simulink model "Simulink"  (R2014a)
settings: Solver=ode45  StartTime=0.0  StopTime=70  RelTol=1e-3
values from neighbouring files (symbols this model uses):
  K = [-4.2029e-03 -3.4474e-01 -1.5683e-01 0.0000 -1.0000e-02]    [Initiallize.m]
  quat0 = attitude(ROCKET.azimth, ROCKET.elevation)'    [Initiallize.m]    (also in RocketSim.m = attitude(azimth, elevation); params.m = attitude(azimth, elevation); params_M3S.m = attitude(ROCKET.azimth, ROCKET.elevation))
  ROCKET = params_rocket()    [Initiallize.m]    (also in params_M3S.m = struct(  'm0', 45247.4,  'Isp', 266,  'g0', 9.80665,  'FT', )
  tau_delta = 0.5    [Initiallize.m]
  Tr = 0.0    (= 0)    [Initiallize.m]
  VWH = [0.0; 0.0; 0.0]    [Initiallize.m]    (also in params.m = [0; 0; 0]; params_M3S.m = [0; 0; 0]; rocket_dynamics.m = [0; 0; 0])
  x0 = [ROCKET.m0; ROCKET.pos0; ROCKET.vel0; quat0; ROCKET.omega0]    [Initiallize.m]    (also in RocketSim.m = [m0; pos0; vel0; quat0; omega0]; params.m = [m0; pos0; vel0; quat0; omega0]; params_M3S.m = [ROCKET.m0; pos0; vel0; quat0; omega0])
undefined symbols (not defined in the file or in its folder): angle0
settings Model: Creator=ikemoto  LastModifiedBy=ikemoto

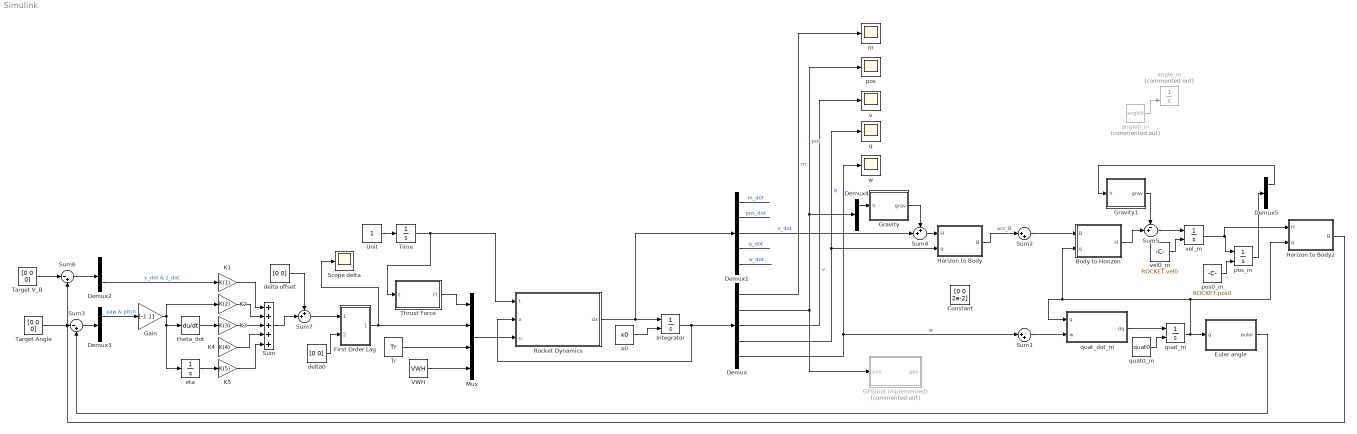
== system Simulink ==
  Body to Horizon : MATLAB Function  TreatAsAtomicUnit=on
  Constant : Constant  Value=[0 0 2e-2]
  Demux : Demux  Outputs=[1 3 3 4 3]
  Demux1 : Demux  Outputs=[1 3 3 4 3]
  Demux2 : Demux  Outputs=[1 2]
  Demux3 : Demux  Outputs=[2 1]
  Demux4 : Demux  Outputs=3
  Demux5 : Demux  Outputs=3
  Euler angle : MATLAB Function  TreatAsAtomicUnit=on
  First Order Lag : Subsystem
  GPS(not implemented) : MATLAB Function  Commented=on  TreatAsAtomicUnit=on
  Gain : Gain  Gain=[-1 1]
  Gravity : MATLAB Function  TreatAsAtomicUnit=on
  Gravity1 : MATLAB Function  TreatAsAtomicUnit=on
  Horizon to Body : MATLAB Function  TreatAsAtomicUnit=on
  Horizon to Body2 : MATLAB Function  TreatAsAtomicUnit=on
  Integrator : Integrator  InitialConditionSource=external  InitialCondition=[4.0 0.0 0.0 0.0 0.0 0.0 0.0 1.0 0.0 0.0 0.0 0.0 0.0 0.0]
  K1 : Gain  Gain=K(1)
  K2 : Gain  Gain=K(2)
  K3 : Gain  Gain=K(3)
  K4 : Gain  Gain=K(4)
  K5 : Gain  Gain=K(5)
  Mux : Mux  Inputs=[1 2 1 3]
  Rocket Dynamics : MATLAB Function  TreatAsAtomicUnit=on
  Scope delta : Scope
      settings: SaveName=ScopeData7
  Sum : Sum  Inputs=+++++
  Sum1 : Sum  Inputs=|++
  Sum2 : Sum  Inputs=|++
  Sum3 : Sum  Inputs=|-+
  Sum4 : Sum  Inputs=++|
  Sum5 : Sum  Inputs=-+|
  Sum6 : Sum  Inputs=|-+
  Sum7 : Sum  Inputs=++|
  Target Angle : Constant  Value=[0 0 0]
  Target V_B : Constant  Value=[0 0 0]
  Thrust Force : MATLAB Function  TreatAsAtomicUnit=on
  Time : Integrator
  Tr : Constant  Value=Tr
  Unit : Constant
  VWH : Constant  Value=VWH
  angle0_m : Constant  Commented=on  Value=angle0
  angle_m : Integrator  Commented=on  InitialConditionSource=external
  delta offset : Constant  Value=[0 0]
  delta0 : Constant  Value=[0 0]
  eta : Integrator
  m : Scope
  pos : Scope
  pos0_m : Constant  Value=ROCKET.pos0
  pos_m : Integrator  InitialConditionSource=external
  q : Scope
      settings: SaveName=ScopeData3
  quat0_m : Constant  Value=quat0
  quat_dot_m : MATLAB Function  TreatAsAtomicUnit=on
  quat_m : Integrator  InitialConditionSource=external
  theta_dot : Derivative
  v : Scope
      settings: SaveName=ScopeData2
  vel0_m : Constant  Value=ROCKET.vel0
  vel_m : Integrator  InitialConditionSource=external
  w : Scope
      settings: SaveName=ScopeData4
  x0 : Constant  Value=x0
  wires:
  Rocket Dynamics/1(dx) -> Demux1/1, Integrator/1
  Integrator/1 -> Rocket Dynamics/2(x), Demux/1
  x0/1 -> Integrator/2
  Demux/1 -> m/1  "m"
  Demux/2 -> pos/1, Demux4/1, GPS(not implemented)/1(pos)  "pos"
  Demux/3 -> v/1  "v"
  Time/1 -> Thrust Force/1(t), Rocket Dynamics/1(t)
  Unit/1 -> Time/1
  Demux1/1 -> ?  "m_dot"
  Demux1/2 -> ?  "pos_dot"
  Demux1/4 -> ?  "q_dot"
  Demux1/5 -> ?  "w_dot"
  Demux/5 -> w/1, Sum1/1  "w"
  Mux/1 -> Rocket Dynamics/3(u)
  VWH/1 -> Mux/4
  Tr/1 -> Mux/3
  vel_m/1 -> Horizon to Body2/1(H), pos_m/1
  eta/1 -> K5/1
  theta_dot/1 -> K3/1
  Gain/1 -> K2/1, eta/1, theta_dot/1
  quat_dot_m/1(dq) -> quat_m/1
  quat0_m/1 -> quat_m/2
  quat_m/1 -> Euler angle/1(q), quat_dot_m/1(q), Body to Horizon/2(q), Horizon to Body2/2(q)
  Thrust Force/1(Ft) -> Mux/1
  Sum1/1 -> quat_dot_m/2(w)
  ? -> Sum1/2  "error"
  ? -> Sum2/2  "error"
  angle0_m/1 -> angle_m/2
  Sum2/1 -> Body to Horizon/1(B)
  vel0_m/1 -> vel_m/2
  pos0_m/1 -> pos_m/2
  Euler angle/1(euler) -> Sum3/2
  Demux2/2 -> K1/1  "y_dot & z_dot"
  K2/1 -> Sum/2
  K1/1 -> Sum/1
  K3/1 -> Sum/3
  K4/1 -> Sum/4
  K5/1 -> Sum/5
  Demux/4 -> q/1, Horizon to Body/2(q)  "q"
  Horizon to Body2/1(B) -> Sum6/2
  Sum3/1 -> Demux3/1
  Target Angle/1 -> Sum3/1
  Demux3/1 -> Gain/1  "yaw & pitch"
  delta0/1 -> First Order Lag/2(delta0)
  First Order Lag/1(delta) -> Scope delta/1, Mux/2
  Horizon to Body/1(B) -> Sum2/1  "acc_B"
  Demux4/1 -> Gravity/1(h)
  Sum5/1 -> vel_m/1
  Body to Horizon/1(H) -> Sum5/2
  Gravity1/1(grav) -> Sum5/1
  pos_m/1 -> Demux5/1
  Demux5/1 -> Gravity1/1(h)
  Sum4/1 -> Horizon to Body/1(H)
  Gravity/1(grav) -> Sum4/1
  Demux1/3 -> Sum4/2  "v_dot"
  Sum6/1 -> Demux2/1
  Target V_B/1 -> Sum6/1
  Sum7/1 -> First Order Lag/1(delta_i)
  Sum/1 -> Sum7/2
  delta offset/1 -> Sum7/1

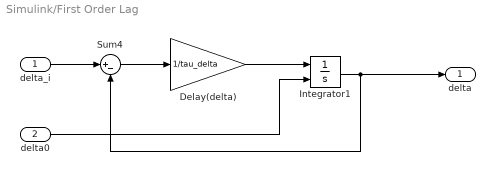
== system Simulink/First Order Lag ==
  delta_i : Inport
  delta0 : Inport  Port=2
  Delay(delta) : Gain  Gain=1/tau_delta
  Integrator1 : Integrator  InitialConditionSource=external  InitialCondition=[4.0 0.0 0.0 0.0 0.0 0.0 0.0 1.0 0.0 0.0 0.0 0.0 0.0 0.0]
  Sum4 : Sum  Inputs=|+-
  delta : Outport
  wires:
  Delay(delta)/1 -> Integrator1/1
  delta0/1 -> Integrator1/2
  Integrator1/1 -> delta/1, Sum4/2
  Sum4/1 -> Delay(delta)/1
  delta_i/1 -> Sum4/1

== matlab function Simulink/GPS(not implemented) ==
  data: pos input; gps output
function gps = GPS_sim(pos)
%#codegen
% 未実装

gps = pos;

== matlab function Simulink/Rocket Dynamics ==
  data: t input size=1; x input size=14; u input size=7; dx output size=14

function dx   = rocket_dynamics_sim( t, x, u)
% t: time 時刻[s]
% x(1): mass 質量[kg]
% x(2): X_H 射点座標位置[m]
% x(3): Y_H 射点座標位置[m]
% x(4): Z_H 射点座標位置[m]
% x(5): VX_H 射点座標対地速度[m/s]
% x(6): VY_H 射点座標対地速度[m/s]
% x(7): VZ_H 射点座標対地速度[m/s]
% x(8): q0 quaternion Body to Horizon[-]
% x(9): q1 quaternion Body to Horizon[-]
% x(10): q2 quaternion Body to Horizon[-]
% x(11): q3 quaternion Body to Horizon[-]
% x(12): omegaX 機体座標系の角速度[rad/s]
% x(13): omegaY 機体座標系の角速度[rad/s]
% x(14): omegaZ 機体座標系の角速度[rad/s]
% u(1): Ft 推力[N]
% u(2): deltaY ヨージンバル角[rad]
% u(3): deltaP ピッチジンバル角[rad]
% u(4): Tr ロール制御トルク[N*m]
% u(5): VWHx 水平座標系における風ベクトル[m/s]
% u(6): VWHy 水平座標系における風ベクトル[m/s]
% u(7): VWHz 水平座標系における風ベクトル[m/s]
% ----
 dx = rocket_dynamics(t,x,u);
end

== matlab function Simulink/quat_dot_m ==
  data: q input; w input; dq output
function dq = deltaquat_sim(q, w)
%#codegen

dq = deltaquat(q, w);
end

== matlab function Simulink/Euler angle ==
  data: q input; euler output
function euler = quat2euler_sim(q)
% QUAT2EULER UEN座標系からの3-2-1の回転でのyaw,pitch,rollのオイラー角
% @param q: UEN座標系から機体座標系への変換クォータニオン (Nx4)
% @return angles: 3-2-1の回転でのyaw, pitch, rollのオイラー角(rad) (Nx3)
%
%   Examples:
%
%   Determine the Euler angles from q = [1 0 1 0]:
%      ea = quat2euler([1 0 1 0])
%
%   Determine the Euler angles from multiple quaternions:
%      q = [1 0 1 0; 1 0.5 0.3 0.1];
%      ea = quat2euler(q)

%#codegen

euler = quat2euler(q');

== matlab function Simulink/Thrust Force ==
  data: t input; Ft output
function Ft = thrust_sim(t)
%#codegen
ROCKET = params_rocket();
Ft = thrust(t, ROCKET.Tend, ROCKET.FT);
end

== matlab function Simulink/Horizon to Body ==
  data: H input; B output; q input
function B = H2B(H, q)
%#codegen

qB = quatmultiply(q, quatmultiply([0 H'], quatconj(q)));
B = qB(2:4)';

== matlab function Simulink/Body to Horizon ==
  data: B input; H output; q input
function H = B2H(B, q)
%#codegen

qH = quatmultiply(quatconj(q), quatmultiply([0 B'], q));
H = qH(2:4)';

== matlab function Simulink/Horizon to Body2 ==
  data: H input; B output; q input
function B = H2B(H, q)
%#codegen

qB = quatmultiply(q, quatmultiply([0 H'], quatconj(q)));
B = qB(2:4)';

== matlab function Simulink/Gravity ==
  data: h input; grav output
function grav = gravity_sim(h)
%#codegen

lat = 35*pi/180;
[gc, gnorth] = gravity(h, lat);
grav = [gc; 0.0; gnorth];

== matlab function Simulink/Gravity1 ==
  data: h input; grav output
function grav = gravity_sim(h)
%#codegen

lat = 35*pi/180;
[gc, gnorth] = gravity(h, lat);
grav = [gc; 0.0; gnorth];
